simulink model "prob2"  (R2020b)
settings: Solver=VariableStepAuto  StartTime=0.0  StopTime=10.0  RelTol=1e-3
values from neighbouring files (symbols this model uses):
  be = 2.0    [data_dict.sldd]
  bv = 1.0    [data_dict.sldd]
  Ie = 1.0    [data_dict.sldd]
  Iv = 5.0    [data_dict.sldd]
settings Model: Creator=nadee  LastModifiedBy=nadee

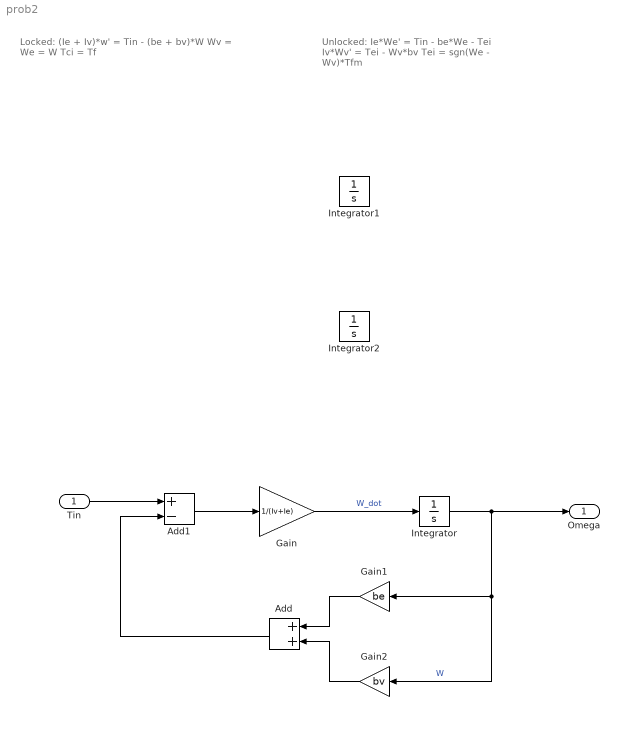
== system prob2 ==
  note: Unlocked:
      | Ie*We' = Tin - be*We - Tei
      | Iv*Wv' = Tei - Wv*bv
      | Tei = sgn(We - Wv)*Tfm
  note: Locked:
      | (Ie + Iv)*w' = Tin - (be + bv)*W
      | Wv = We = W
      | Tci = Tf
  Tin : Inport
  Add : Sum
  Add1 : Sum  Inputs=+-
  Gain : Gain  Gain=1/(Iv+Ie)
  Gain1 : Gain  Gain=be
  Gain2 : Gain  Gain=bv
  Integrator : Integrator
  Integrator1 : Integrator
  Integrator2 : Integrator
  Omega : Outport
  wires:
  Gain/1 -> Integrator/1  "W_dot"
  Add1/1 -> Gain/1
  Add/1 -> Add1/2
  Tin/1 -> Add1/1
  Gain2/1 -> Add/2
  Gain1/1 -> Add/1
  Integrator/1 -> Gain2/1, Gain1/1, Omega/1  "W"
